simulink model "challenge1_integralAction"  (R2025a)
settings: Solver=ode45  StartTime=0.0  StopTime=3  RelTol=1e-3
undefined symbols (not defined in the file): degs2rpm, delta_c, den_Hi, K_g, KI, mot, Nu, num_Hi, Nx, rpm2rads, sens, w_c
libraries: simulink x1
settings Model: Creator=ester  LastModifiedBy=ester

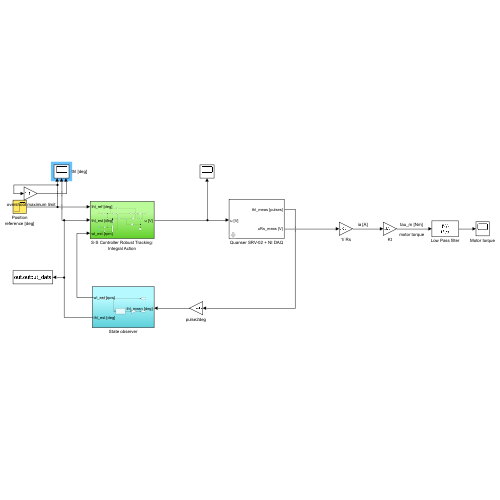
[thumbnail: Simulink's stored preview of the top-level diagram]
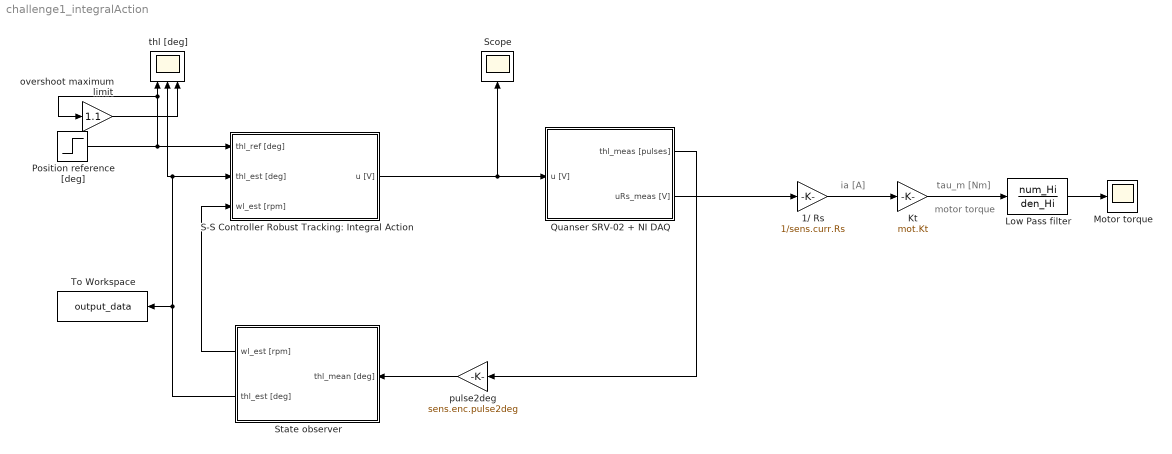
== system challenge1_integralAction ==
  note: motor torque
  note: tau_m [Nm]
  note: ia [A]
  " overshoot maximum limit" : Gain  Gain=1.1
  1/ Rs : Gain  Gain=1/sens.curr.Rs
  Kt : Gain  Gain=mot.Kt
  Low Pass filter : TransferFcn  Numerator=num_Hi  Denominator=den_Hi
  Motor torque : Scope
      settings: ActiveDisplayYMinimum=-0.010577411968592633  ActiveDisplayYMaximum=0.011875949900729958  DataLoggingVariableName=ScopeData4
  Position reference [deg] : Step  Time=0  After=70  SampleTime=0  ZeroCross=off
  Quanser SRV-02 + NI DAQ : Subsystem  mask(Quanser SRV-02 (with inertial load) + NI DAQ){Ts=0.001, fricType=Coulomb + viscous}
      mask prompts: Ts "NI DAQ Sample Time:"; fricType "Friction model"
      mask help: Quanser SRV-02 (with inertial load) + NI DAQ model.
      mask init:
      | %%  Sensors data
      | 
      | %   shunt resistor
      | sens.curr.Rs = 0.5;                         %   resistance [Ohm]   
      | sens.curr.uRs_std = 0.01;                   %   voltage noise standard dev [V]                           
      | sens.curr.uRs_var = sens.curr.uRs_std^2;	%   voltage noise variance [V^2]
      | 
      | %   Hewlett-Packard HEDS-5540#A06 optical encoder
      | sens.enc.ppr = 500*4;                       %   pulses per rotation
      | sens.enc.pulse2deg = 360/sens.enc.ppr;      %   [pulses] -> [deg]
      | sens.enc.pulse2rad = 2*pi/sens.enc.ppr;     %   [pulses] -> [rad]
      | sens.enc.deg2pulse = sens.enc.ppr/360;      %   [deg] -> [pulses]
      | sens.enc.rad2pulse = sens.enc.ppr/2/pi;     %   [rad] -> [pulses]
      | 
      | 
      | %%  Data acquisition board (daq) data
      | 
      | %   NI PCI-6221 DAC data
      | daq.dac.bits = 16;                                  %   resolution (bits)
      | daq.dac.fs   = 10;                                  %   full scale 
      | daq.dac.q    = 2*daq.dac.fs/(2^daq.dac.bits-1);     %	quantization
      | 
      | %   NI PCI-6221 ADC data
      | daq.adc.bits = 16;                                  %   resolution (bits)
      | daq.adc.fs   = 10;                                  %   full scale (as set in SLDRT Analog Input block)
      | daq.adc.q    = 2*daq.adc.fs/(2^daq.adc.bits-1);     %   quantization
      mask Help:
      | Riccardo Antonello (antonello@dei.unipd.it)
      | 
      | April 24, 2020
      | 
      | Dept. of Information Engineering, University of Padova
      mask TypeOptions fricType: Coulomb + viscous | Karnopp
  S-S Controller Robust Tracking: Integral Action : Subsystem
  Scope : Scope
      settings: ActiveDisplayYMinimum=-1  ActiveDisplayYMaximum=1
  State observer : Subsystem
  To Workspace : ToWorkspace  VariableName=output_data  SaveFormat=Timeseries  SampleTime=-1
  pulse2deg : Gain  Gain=sens.enc.pulse2deg
  thl [deg] : Scope  NumInputPorts=3
      settings: ActiveDisplayYMinimum=-9.6249999999999982  ActiveDisplayYMaximum=86.625
  wires:
  State observer/2(thl_est [deg]) -> To Workspace/1, thl [deg]/2, S-S Controller Robust Tracking: Integral Action/2(thl_est [deg])
  State observer/1(wl_est [rpm]) -> S-S Controller Robust Tracking: Integral Action/3(wl_est [rpm])
  pulse2deg/1 -> State observer/1(thl_mean [deg])
  Position reference [deg]/1 -> S-S Controller Robust Tracking: Integral Action/1(thl_ref [deg]), " overshoot maximum limit"/1, thl [deg]/1
  S-S Controller Robust Tracking: Integral Action/1(u [V]) -> Scope/1, Quanser SRV-02 + NI DAQ/1(u [V])
  Quanser SRV-02 + NI DAQ/1(thl_meas [pulses]) -> pulse2deg/1
  Kt/1 -> Low Pass filter/1
  1/ Rs/1 -> Kt/1
  Quanser SRV-02 + NI DAQ/2(uRs_meas [V]) -> 1/ Rs/1
  Low Pass filter/1 -> Motor torque/1
  " overshoot maximum limit"/1 -> thl [deg]/3

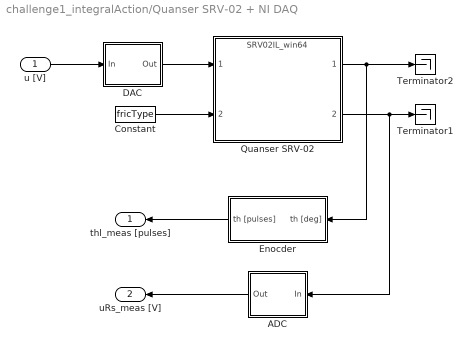
== system challenge1_integralAction/Quanser SRV-02 + NI DAQ ==
  u [V] : Inport
  ADC : Subsystem
  Constant : Constant  Value=fricType
  DAC : Subsystem
  Enocder : Subsystem
  Quanser SRV-02 : ModelReference  ModelNameDialog=SRV02IL_win64.slxp  ModelReferenceVersion=1.44  CopyOfModelProtected=on
  Terminator1 : Terminator
  Terminator2 : Terminator
  thl_meas [pulses] : Outport
  uRs_meas [V] : Outport  Port=2
  wires:
  Enocder/1(th [pulses]) -> thl_meas [pulses]/1
  ADC/1(Out) -> uRs_meas [V]/1
  DAC/1(Out) -> Quanser SRV-02/1
  Quanser SRV-02/2 -> ADC/1(In), Terminator1/1
  u [V]/1 -> DAC/1(In)
  Quanser SRV-02/1 -> Enocder/1(th [deg]), Terminator2/1
  Constant/1 -> Quanser SRV-02/2

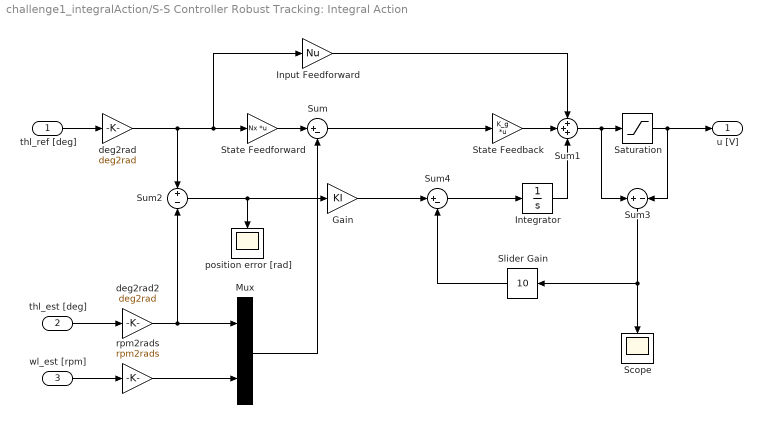
== system challenge1_integralAction/S-S Controller Robust Tracking: Integral Action ==
  thl_ref [deg] : Inport
  thl_est [deg] : Inport  Port=2
  wl_est [rpm] : Inport  Port=3
  Gain : Gain  Gain=KI
  Input Feedforward : Gain  Gain=Nu
  Integrator : Integrator
  Mux : Mux  Inputs=2
  Saturation : Saturate  UpperLimit=10  LowerLimit=-10  ZeroCross=off
  Scope : Scope
      settings: ActiveDisplayYMinimum=-2.5760390517348313  ActiveDisplayYMaximum=48.6610372415814  DataLoggingVariableName=ScopeData3
  Slider Gain : simulink/Math Operations/Slider Gain  gain=10  low=0  high=50
  State Feedback : Gain  Gain=K_g  Multiplication=Matrix(K*u)
  State Feedforward : Gain  Gain=Nx  Multiplication=Matrix(K*u)
  Sum : Sum  Inputs=|+-
  Sum1 : Sum  Inputs=+++
  Sum2 : Sum  Inputs=+-
  Sum3 : Sum  Inputs=+|-
  Sum4 : Sum  Inputs=|+-
  deg2rad : Gain  Gain=deg2rad
  deg2rad2 : Gain  Gain=deg2rad
  position error [rad] : Scope
      settings: ActiveDisplayYMinimum=-1.27025  ActiveDisplayYMaximum=2.46824  DataLoggingVariableName=ScopeData2
  rpm2rads : Gain  Gain=rpm2rads
  u [V] : Outport
  wires:
  Saturation/1 -> Sum3/2, u [V]/1
  wl_est [rpm]/1 -> rpm2rads/1
  thl_ref [deg]/1 -> deg2rad/1
  Sum1/1 -> Sum3/1, Saturation/1
  deg2rad/1 -> State Feedforward/1, Input Feedforward/1, Sum2/1
  Mux/1 -> Sum/2
  Input Feedforward/1 -> Sum1/1
  Sum/1 -> State Feedback/1
  State Feedforward/1 -> Sum/1
  rpm2rads/1 -> Mux/2
  thl_est [deg]/1 -> deg2rad2/1
  deg2rad2/1 -> Sum2/2, Mux/1
  State Feedback/1 -> Sum1/2
  Integrator/1 -> Sum1/3
  Sum2/1 -> Gain/1, position error [rad]/1
  Sum3/1 -> Slider Gain/1, Scope/1
  Gain/1 -> Sum4/1
  Sum4/1 -> Integrator/1
  Slider Gain/1 -> Sum4/2

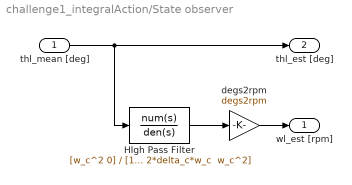
== system challenge1_integralAction/State observer ==
  thl_mean [deg] : Inport
  HIgh Pass Filter : TransferFcn  Numerator=[w_c^2 0]  Denominator="[1 2*delta_c*w_c  w_c^2]"
  degs2rpm : Gain  Gain=degs2rpm
  wl_est [rpm] : Outport
  thl_est [deg] : Outport  Port=2
  wires:
  thl_mean [deg]/1 -> HIgh Pass Filter/1, thl_est [deg]/1
  HIgh Pass Filter/1 -> degs2rpm/1
  degs2rpm/1 -> wl_est [rpm]/1

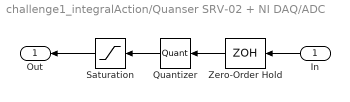
== system challenge1_integralAction/Quanser SRV-02 + NI DAQ/ADC ==
  In : Inport
  Quantizer : Quantizer  QuantizationInterval=daq.adc.q
  Saturation : Saturate  UpperLimit=daq.adc.fs  LowerLimit=-daq.adc.fs
  Zero-Order Hold : ZeroOrderHold  SampleTime=Ts
  Out : Outport
  wires:
  Saturation/1 -> Out/1
  In/1 -> Zero-Order Hold/1
  Quantizer/1 -> Saturation/1
  Zero-Order Hold/1 -> Quantizer/1

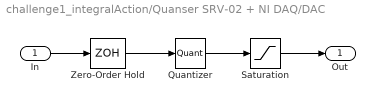
== system challenge1_integralAction/Quanser SRV-02 + NI DAQ/DAC ==
  In : Inport
  Quantizer : Quantizer  QuantizationInterval=daq.dac.q
  Saturation : Saturate  UpperLimit=daq.dac.fs  LowerLimit=-daq.dac.fs
  Zero-Order Hold : ZeroOrderHold  SampleTime=Ts
  Out : Outport
  wires:
  Quantizer/1 -> Saturation/1
  In/1 -> Zero-Order Hold/1
  Zero-Order Hold/1 -> Quantizer/1
  Saturation/1 -> Out/1

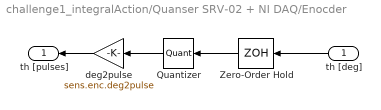
== system challenge1_integralAction/Quanser SRV-02 + NI DAQ/Enocder ==
  th [deg] : Inport
  Quantizer : Quantizer  QuantizationInterval=sens.enc.pulse2deg
  Zero-Order Hold : ZeroOrderHold  SampleTime=Ts
  deg2pulse : Gain  Gain=sens.enc.deg2pulse
  th [pulses] : Outport
  wires:
  Quantizer/1 -> deg2pulse/1
  th [deg]/1 -> Zero-Order Hold/1
  Zero-Order Hold/1 -> Quantizer/1
  deg2pulse/1 -> th [pulses]/1
